simulink model "simscape_automatic_R2024a"  (R2024a)
settings: Solver=ode15s  StartTime=0.0  StopTime=inf  FixedStep=timestep
values from neighbouring files (symbols this model uses):
  timestep = 0.5    [design_details.m]
undefined symbols (not defined in the file or in its folder): CONNECTED, DEFUEL_MODE, DISCONNECT, DISCONNECTED, REFUEL_MODE
settings Model: PacingRate=0.100000  TunableVars=AC_mode_data,AC_tank_cross_sectional_area,AC_tank_radius,AC_tank_surface_area,AC_tank_vol_limit,AC_tank_volume,AC_tank_weight,AC_wall_thickness,Ambient_temp,Equivalent_battery_mass,GH2_conductivity,Generator_efficiency,H2Tables,H2_energy_density,Initial_AC_LH2_frac,Initial_AC_Tank_Gas_Temp,Initial_AC_Tank_Liquid_Temp,Initial_AC_tank_pressure,Initial_temp,LH2_conductivity,LH2_density,LH2_density_table,Required_energy,Temp_vector,engine_feed_pipe_inner_area,engine_feed_pipe_inner_diameter,engine_feed_pipe_outer_area,engine_feed_pipe_outer_diameter,engine_feed_valve_discharge_ratio,engine_feed_valve_orifice_area,engine_feed_valve_orifice_radius,hose_length,hose_thermal_conductivity,initial_hose_p,liquid_supply_SOV_leak_frac,m_LH2,mass_flow_rate,mass_per_length_engine_feed,mass_per_length_return,mass_per_length_supply,max_pressure,max_stress,phase,pipe_thermal_conductivity,pressure_vector,radiation_constant,refuel_time,return_pipe_inner_area,return_pipe_inner_diameter,return_pipe_outer_area,return_pipe_outer_diameter,return_valve_discharge_ratio,return_valve_orifice_area,return_valve_orifice_radius,short_pressure_vector,short_temp_vector,steel_conductivity,steel_density,steel_emmissitivity,steel_heat_capacity,stopTime,supply_pipe_inner_area,supply_pipe_inner_diameter,supply_pipe_outer_area,supply_pipe_outer_diameter,supply_valve_discharge_ratio,supply_valve_orifice_area,supply_valve_orifice_radius,time_array,timestep,u_max_gas,u_min_liquid,valve_diameter_vector,valve_laminar_p_ratio,wall_thickness,AC_return_valve_discharge_coeff,AC_return_valve_inner_diameter,AC_return_valve_laminar_p_ratio,AC_return_valve_leakage,AC_return_valve_orifice_area,AC_return_valve_port_inner_area,AC_return_valve_port_inner_diameter,AC_supply_valve_discharge_coeff,AC_supply_valve_inner_diameter,AC_supply_valve_laminar_p_ratio,AC_supply_valve_leakage,AC_supply_valve_orifice_area,AC_supply_valve_port_inner_area,AC_supply_valve_port_inner_diameter,GS_return_valve_discharge_coeff,GS_return_valve_inner_diameter,GS_return_valve_laminar_p_ratio,GS_return_valve_leakage,GS_return_valve_orifice_area,GS_return_valve_port_inner_area,GS_return_valve_port_inner_diameter,GS_supply_valve_discharge_coeff,GS_supply_valve_inner_diameter,GS_supply_valve_laminar_p_ratio,GS_supply_valve_leakage,GS_supply_valve_orifice_area,GS_supply_valve_port_inner_area,GS_supply_valve_port_inner_diameter,LH2_prop_valve_discharge_coeff,LH2_prop_valve_inner_diameter,LH2_prop_valve_laminar_p_ratio,LH2_prop_valve_leakage,LH2_prop_valve_orifice_area,LH2_prop_valve_port_inner_area,LH2_prop_valve_port_inner_diameter,Return_gas_prop_valve_discharge_coeff,Return_gas_prop_valve_inner_diameter,Return_gas_prop_valve_laminar_p_ratio,Return_gas_prop_valve_leakage,Return_gas_prop_valve_orifice_area,Return_gas_prop_valve_port_inner_area,Return_gas_prop_valve_port_inner_diameter,return_coupling_discharge_coeff,return_coupling_port_inner_area,return_coupling_port_inner_diameter,return_coupling_valve_inner_diameter,return_coupling_valve_laminar_p_ratio,return_coupling_valve_leakage,return_coupling_valve_orifice_area,supply_coupling_discharge_coeff,supply_coupling_port_inner_area,supply_coupling_port_inner_diameter,supply_coupling_valve_inner_diameter,supply_coupling_valve_laminar_p_ratio,supply_coupling_valve_leakage,supply_coupling_valve_orifice_area,AC_bypass_line_port_inner_area,AC_bypass_line_port_inner_diameter,AC_bypass_line_port_outer_diameter,AC_bypass_pipe_length,AC_engine_feed_pipe_length,AC_engine_feed_port_inner_area,AC_engine_feed_port_inner_diameter,AC_engine_feed_port_outer_diameter,AC_engine_valve_discharge_coeff,AC_engine_valve_inner_diameter,AC_engine_valve_laminar_p_ratio,AC_engine_valve_leakage,AC_engine_valve_orifice_area,AC_return_line_port_inner_area,AC_return_line_port_inner_diameter,AC_return_line_port_outer_diameter,AC_return_pipe_length,AC_supply_line_port_inner_area,AC_supply_line_port_inner_diameter,AC_supply_line_port_outer_diameter,AC_supply_pipe_length,AC_vent_line_port_inner_area,AC_vent_line_port_inner_diameter,AC_vent_valve_discharge_coeff,AC_vent_valve_orifice_area,AC_vent_valve_orifice_inner_diameter,Gas_prop_valve_discharge_coeff,Gas_prop_valve_inner_diameter,Gas_prop_valve_laminar_p_ratio,Gas_prop_valve_leakage,Gas_prop_valve_orifice_area,mass_per_length_bypass,return_valve_orifice_diameter,supply_valve_orifice_diameter,thermal_mass_per_length_bypass,thermal_mass_per_length_engine_feed,thermal_mass_per_length_return,thermal_mass_per_length_supply,ABORT_MODE,AC_tank_liquid_heat_transfer_coeff,AC_tank_vapour_heat_transfer_coeff,CHILLDOWN,CLOSE,CONNECTED,DEFUEL,DEFUEL_MODE,DISCONNECT,DISCONNECTED,FEED,GS_vent_cracking_delta_P,GS_vent_discharge_coeff,GS_vent_open_delta_P,Gas_prop_valve_gain,Gas_prop_valve_stroke,IDLE,LH2_prop_valve_gain,LH2_prop_valve_stroke,OPEN,OVEREFILL,PID_timestep,REFUEL,REFUEL_MODE,Return_gas_prop_valve_gain,Return_gas_prop_valve_min_open,Return_gas_prop_valve_stroke,WARMUP,i,tf_delay,vent_tf_delay  TunableVarsStorageClass=Auto,Auto,Auto,Auto,Auto,Auto,Auto,Auto,Auto,Auto,Auto,Auto,Auto,Auto,Auto,Auto,Auto,Auto,Auto,Auto,Auto,Auto,Auto,Auto,Auto,Auto,Auto,Auto,Auto,Auto,Auto,Auto,Auto,Auto,Auto,Auto,Auto,Auto,Auto,Auto,Auto,Auto,Auto,Auto,Auto,Auto,Auto,Auto,Auto,Auto,Auto,Auto,Auto,Auto,Auto,Auto,Auto,Auto,Auto,Auto,Auto,Auto,Auto,Auto,Auto,Auto,Auto,Auto,Auto,Auto,Auto,Auto,Auto,Auto,Auto,Auto,Auto,Auto,Auto,Auto,Auto,Auto,Auto,Auto,Auto,Auto,Auto,Auto,Auto,Auto,Auto,Auto,Auto,Auto,Auto,Auto,Auto,Auto,Auto,Auto,Auto,Auto,Auto,Auto,Auto,Auto,Auto,Auto,Auto,Auto,Auto,Auto,Auto,Auto,Auto,Auto,Auto,Auto,Auto,Auto,Auto,Auto,Auto,Auto,Auto,Auto,Auto,Auto,Auto,Auto,Auto,Auto,Auto,Auto,Auto,Auto,Auto,Auto,Auto,Auto,Auto,Auto,Auto,Auto,Auto,Auto,Auto,Auto,Auto,Auto,Auto,Auto,Auto,Auto,Auto,Auto,Auto,Auto,Auto,Auto,Auto,Auto,Auto,Auto,Auto,Auto,Auto,Auto,Auto,Auto,Auto,Auto,Auto,Auto,Auto,Auto,Auto,Auto,Auto,Auto,Auto,Auto,Auto,Auto,Auto,Auto,Auto,Auto,Auto,Auto,Auto,Auto,Auto,Auto,Auto,Auto,Auto,Auto,Auto,Auto  TunableVarsTypeQualifier=,,,,,,,,,,,,,,,,,,,,,,,,,,,,,,,,,,,,,,,,,,,,,,,,,,,,,,,,,,,,,,,,,,,,,,,,,,,,,,,,,,,,,,,,,,,,,,,,,,,,,,,,,,,,,,,,,,,,,,,,,,,,,,,,,,,,,,,,,,,,,,,,,,,,,,,,,,,,,,,,,,,,,,,,,,,,,,,,,,,,,,,,,,,,,,,,,,,,,,,  Creator=MW  LastModifiedBy=MW
settings SolverCC: MaxConsecutiveMinStep=3  DaesscMode=Robust  SolverResetMethod=Robust
settings DataIOCC: ReturnWorkspaceOutputsName=tpe7319d77_74b4_4e39_b21d_406e30cb87cb
settings ModelReferenceCC: UpdateModelReferenceTargets=IfOutOfDate
settings SFSimCC: SFSimEcho=off  SimTargetLang=C++  GPUAcceleration=on  SimDLTargetLibrary=cudnn
settings SimscapeCC: SimscapeNominalValues="[{\"value\":\"1\",\"unit\":\"A\"},{\"value\":\"0.3\",\"unit\":\"bar\"},{\"value\":\"1\",\"unit\":\"cm^2\"},{\"value\":\"1\",\"unit\":\"cm^3/s\"},{\"value\":\"1\",\"unit\":\"kJ/kg\"},{\"value\":\"1\",\"unit\":\"kW\"},{\"value\":\"1\",\"unit\":\"l\"},{\"value\":\"1\",\"unit\":\"N\"},{\"value\":\"1\",\"unit\":\"N*m\"},{\"value\":\"1\",\"unit\":\"V\"}]"  SimscapeLogType=all  SimscapeLogSimulationStatistics=on  SimscapeLogLimitData=off

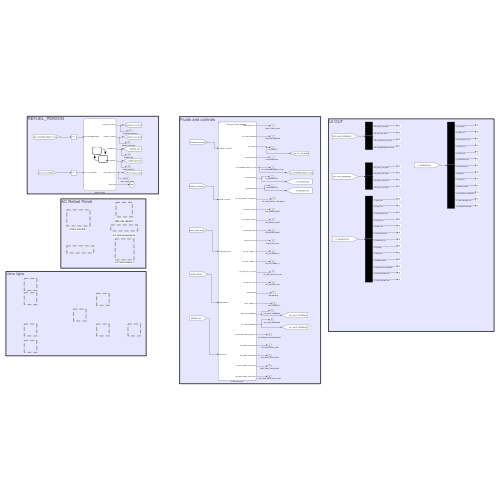
[thumbnail: Simulink's stored preview of the top-level diagram]
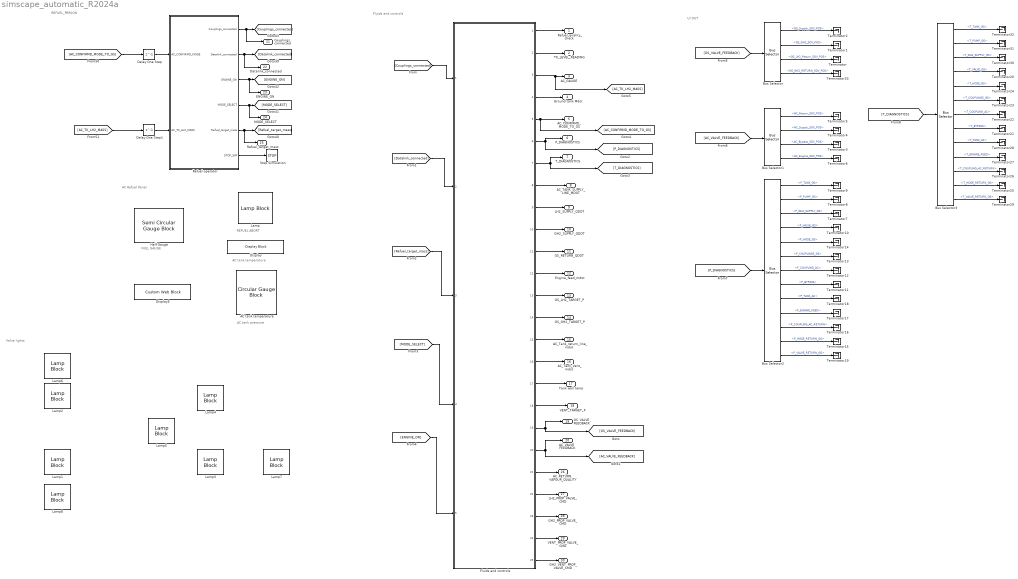
== system simscape_automatic_R2024a ==
  note: REFUEL ABORT
  note: AC tank pressure
  note: AC Refuel Panel
  note: AC tank temperature
  note: REFUEL_PERSON
  note: FUEL GAUGE
  note: UI OUT
  note: Valve lights
  note: Fluids and controls
  AC tank temperature : CircularGaugeBlock  LabelPosition=Hide  ScaleMax=0.7
  Bus Selector : BusSelector  OutputSignals=GS_Supply_SOV_POS,GS_GH2_SOV_POS,GS_LH2_Return_SOV_POS,GS_GH2_RETURN_SOV_POS
  Bus Selector1 : BusSelector  OutputSignals=AC_Return_SOV_POS,AC_Supply_SOV_POS,AC_Bypass_SOV_POS,AC_Engine_SOV_POS
  Bus Selector2 : BusSelector  OutputSignals=P_TANK_GS,P_PUMP_GS,P_GH2_SUPPLY_GS,P_VALVE_GS,P_HOSE_GS,P_COUPLINGS_GS,P_COUPLING_AC,P_BYPASS,P_TANK_AC,P_ENGINE_FEED,P_COUPLING_AC_RETURN,P_HOSE_RETURN_GS,P_VALVE_RETURN_GS
  Bus Selector3 : BusSelector  OutputSignals=T_TANK_GS,T_PUMP_GS,T_GH2_SUPPLY_GS,T_VALVE_GS,T_HOSE_GS,T_COUPLINGS_GS,T_COUPLING_AC,T_BYPASS,T_TANK_AC,T_ENGINE_FEED,T_COUPLING_AC_RETURN,T_HOSE_RETURN_GS,T_VALVE_RETURN_GS
  Delay One Step : Delay  DelayLength=1
  Delay One Step1 : Delay  DelayLength=1
  Display : DisplayBlock  LabelPosition=Hide  Transparency=1
  Display5 : CustomWebBlock  LabelPosition=Hide  ShowInitialText=on  Configuration="{\"components\":[{\"name\":\"DisplayComponent\",\"settings\":{\"bold\":false,\"font\":\"DSEG7 Classic\",\"fontColor\":[255,255,200],\"fontSize\":\"14\",\"format\":\"short\",\"formatString\":\"%d\",\"italic\":false,\"position\":[0,0,1,1],\"underline\":false}},{\"name\":\"BackgroundImageComponent\",\"settings\":{\"image\":{\"size\":[300,80],\"src\":\"data:image\\/svg+xml;base64,PHN2ZyBpZD0iZnJhbWUiIHhtbG5zPSJodHRwOi8vd3d3LnczLm9yZy8yMDAwL3N2ZyIgeG1sbnM6eGxpbms9Imh0dHA6Ly93d3cudzMub3JnLzE5OTkveGxpbmsiIHZpZXdCb3g9IjAgMCAzODAgMTAxIj48ZGVmcz48c3R5bGU+LmNscy0xe2ZpbGw6IzAwMmI0Mjt9LmNscy0ye2ZpbGw6IzQyNzA4Mjt9LmNscy0ze2ZpbGw6dXJsKCNyYWRpYWwtZ3JhZGllbnQpO308L3N0eWxlPjxyYWRpYWxHcmFkaWVudCBpZD0icmFkaWFsLWdyYWRpZW50IiBjeD0iMTkwIiBjeT0iNTAuNSIgcj0iMjY5LjIxIiBncmFkaWVudFVuaXRzPSJ1c2VyU3BhY2VPblVzZSI+PHN0b3Agb2Zmc2V0PSIwLjAxIiBzdG9wLWNvbG9yPSIjM2U0ZjU4Ii8+PHN0b3Agb2Zmc2V0PSIwLjA2IiBzdG9wLWNvbG9yPSIjNDQ1NzYxIi8+PHN0b3Agb2Zmc2V0PSIwLjE1IiBzdG9wLWNvbG9yPSIjNTU2YTc2Ii8+PHN0b3Agb2Zmc2V0PSIwLjI1IiBzdG9wLWNvbG9yPSIjNmQ4ODk1Ii8+PHN0b3Agb2Zmc2V0PSIwLjM4IiBzdG9wLWNvbG9yPSIjOGZiMmMzIi8+PHN0b3Agb2Zmc2V0PSIwLjUyIiBzdG9wLWNvbG9yPSIjYjZlNGZhIi8+PHN0b3Agb2Zmc2V0PSIxIiBzdG9wLWNvbG9yPSIjMTU0NjU3Ii8+PC9yYWRpYWxHcmFkaWVudD48L2RlZnM+PGcgaWQ9IkxheWVyXzIiIGRhdGEtbmFtZT0iTGF5ZXIgMiI+PGcgaWQ9IkxheWVyXzEtMiIgZGF0YS1uYW1lPSJMYXllciAxLTIiPjxyZWN0IGlkPSJyZWN0MTAzNiIgY2xhc3M9ImNscy0xIiB4PSIxMSIgeT0iMTEiIHdpZHRoPSIzNTgiIGhlaWdodD0iNzkiLz48cGF0aCBpZD0icGF0aDEwMzgiIGNsYXNzPSJjbHMtMiIgZD0iTTgsOFY5M0gzNzJWOFpNMzY5LDkwSDExVjExSDM2OVoiLz48cGF0aCBpZD0icGF0aDEwNDAiIGNsYXNzPSJjbHMtMyIgZD0iTTAsMFYxMDFIMzgwVjBaTTM3Miw5M0g4VjhIMzcyWiIvPjwvZz48L2c+PC9zdmc+\",\"srcOrientation\":\"Right\"},\"position\":[0,0,1,1],\"scaleMode\":\"0\"}},{\"name\":\"ForegroundImageComponent\",\"settings\":{\"angle\":0,\"image\":{\"size\":[0,0],\"src\":\"default\"},\"isForeground\":1,\"position\":[0,0,1,1],\"scaleMode\":\"0\"}}],\"settings\":{\"BindingType\":\"signal\",\"aspectRatio\":1.032258064516129,\"backgroundColor\":[0,0,0,\"1\"],\"backgroundOffset\":0.14,\"backgroundOpacity\":1,\"fixedAspectRatio\":\"on\",\"showBackgroundColor\":false,\"value\":0,\"version\":\"R2023b\"},\"type\":\"Display\"}"
  Fluids and controls : Subsystem  ReferencedSubsystem=fluids_and_control_subsystem
  Half Gauge : SemiCircularGaugeBlock  ScaleMax=35
  Lamp{,1..8} (9 alike) : LampBlock  LabelPosition=Hide
  Refuel operator : Stateflow chart  TreatAsAtomicUnit=on  SystemSampleTime=timestep
  Stop Simulation : Stop
  Terminator{,1..33} (34 alike) : Terminator
  Refuel_quality_check : Outport
  TK_LEVEL_READING : Outport  Port=2
  AC_GAUGE : Outport  Port=3
  Ground tank Mdot : Outport  Port=4
  AC_CONFIRMD_MODE_TO_GS : Outport  Port=5
  P_DIAGNOSTICS : Outport  Port=6
  T_DIAGNOSTICS : Outport  Port=7
  AC_TANK_SUPPLY_LINE_MDOT : Outport  Port=8
  LH2_SUPPLY_QDOT : Outport  Port=9
  GH2_SUPPLY_QDOT : Outport  Port=10
  GS_RETURN_QDOT : Outport  Port=11
  Engine_feed_mdot : Outport  Port=12
  GS_LH2_TARGET_P : Outport  Port=13
  GS_GH2_TARGET_P : Outport  Port=14
  AC_Tank_return_line_mdot : Outport  Port=15
  AC_Tank_Vent_mdot : Outport  Port=16
  Tank wall temp : Outport  Port=17
  VENT_TARGET_P : Outport  Port=18
  GS_VALVE_FEEDBACK : Outport  Port=19
  AC_VALVE_FEEDBACK : Outport  Port=20
  Couplings_connected : Outport  Port=21
  Datalink_connected : Outport  Port=22
  ENGINE_ON : Outport  Port=23
  MODE_SELECT : Outport  Port=24
  Refuel_target_mass : Outport  Port=25
  AC_RETURN_VAPOUR_QUALITY : Outport  Port=26
  LH2_PROP_VALVE_CMD : Outport  Port=27
  GH2_PROP_VALVE_CMD : Outport  Port=28
  VENT_PROP_VALVE_CMD : Outport  Port=29
  GH2_VENT_PROP_VALVE_CMD : Outport  Port=30
  wires:
  Refuel operator/1(Couplings_connected) -> Couplings_connected/1, [Couplings_connected]
  Refuel operator/2(Datalink_connected) -> Datalink_connected/1, [Datalink_connected]
  Refuel operator/4(MODE_SELECT) -> MODE_SELECT/1, [MODE_SELECT]
  Refuel operator/3(ENGINE_ON) -> ENGINE_ON/1, [ENGINE_ON]
  Refuel operator/5(Refuel_target_mass) -> Refuel_target_mass/1, [Refuel_target_mass]
  [AC_CONFIRMD_MODE_TO_GS] -> Delay One Step/1
  Delay One Step/1 -> Refuel operator/1(AC_CONFIRMD_MODE)
  [AC_TK_LH2_MASS] -> Delay One Step1/1
  Delay One Step1/1 -> Refuel operator/2(AC_TK_LH2_MASS)
  Refuel operator/6(STOP_SIM) -> Stop Simulation/1
  [T_DIAGNOSTICS] -> Bus Selector3/1
  Bus Selector3/3 -> Terminator30/1  "<T_GH2_SUPPLY_GS>"
  Bus Selector/1 -> Terminator2/1  "<GS_Supply_SOV_POS>"
  Bus Selector3/2 -> Terminator31/1  "<T_PUMP_GS>"
  Bus Selector3/12 -> Terminator25/1  "<T_HOSE_RETURN_GS>"
  Bus Selector2/9 -> Terminator18/1  "<P_TANK_AC>"
  Bus Selector3/11 -> Terminator26/1  "<T_COUPLING_AC_RETURN>"
  Bus Selector3/4 -> Terminator20/1  "<T_VALVE_GS>"
  Bus Selector/3 -> Terminator/1  "<GS_LH2_Return_SOV_POS>"
  Bus Selector3/5 -> Terminator24/1  "<T_HOSE_GS>"
  Bus Selector3/6 -> Terminator23/1  "<T_COUPLINGS_GS>"
  [GS_VALVE_FEEDBACK] -> Bus Selector/1
  Bus Selector2/5 -> Terminator14/1  "<P_HOSE_GS>"
  Bus Selector2/3 -> Terminator7/1  "<P_GH2_SUPPLY_GS>"
  Bus Selector1/1 -> Terminator5/1  "<AC_Return_SOV_POS>"
  Bus Selector2/7 -> Terminator12/1  "<P_COUPLING_AC>"
  Bus Selector3/9 -> Terminator28/1  "<T_TANK_AC>"
  Bus Selector3/1 -> Terminator32/1  "<T_TANK_GS>"
  Bus Selector2/13 -> Terminator19/1  "<P_VALVE_RETURN_GS>"
  Bus Selector3/10 -> Terminator27/1  "<T_ENGINE_FEED>"
  Bus Selector2/12 -> Terminator15/1  "<P_HOSE_RETURN_GS>"
  Bus Selector1/4 -> Terminator6/1  "<AC_Engine_SOV_POS>"
  Bus Selector2/6 -> Terminator13/1  "<P_COUPLINGS_GS>"
  [P_DIAGNOSTICS] -> Bus Selector2/1
  Bus Selector2/4 -> Terminator10/1  "<P_VALVE_GS>"
  Bus Selector2/11 -> Terminator16/1  "<P_COUPLING_AC_RETURN>"
  Bus Selector3/13 -> Terminator29/1  "<T_VALVE_RETURN_GS>"
  Bus Selector2/2 -> Terminator8/1  "<P_PUMP_GS>"
  [AC_VALVE_FEEDBACK] -> Bus Selector1/1
  Bus Selector1/2 -> Terminator4/1  "<AC_Supply_SOV_POS>"
  Bus Selector/2 -> Terminator1/1  "<GS_GH2_SOV_POS>"
  Bus Selector1/3 -> Terminator3/1  "<AC_Bypass_SOV_POS>"
  Bus Selector2/8 -> Terminator11/1  "<P_BYPASS>"
  Bus Selector3/7 -> Terminator22/1  "<T_COUPLING_AC>"
  Bus Selector2/10 -> Terminator17/1  "<P_ENGINE_FEED>"
  Bus Selector2/1 -> Terminator9/1  "<P_TANK_GS>"
  Bus Selector3/8 -> Terminator21/1  "<T_BYPASS>"
  Fluids and controls/6 -> P_DIAGNOSTICS/1, [P_DIAGNOSTICS]
  Fluids and controls/16 -> AC_Tank_Vent_mdot/1
  Fluids and controls/3 -> [AC_TK_LH2_MASS], AC_GAUGE/1
  [Datalink_connected] -> Fluids and controls/2
  Fluids and controls/9 -> LH2_SUPPLY_QDOT/1
  Fluids and controls/11 -> GS_RETURN_QDOT/1
  Fluids and controls/2 -> TK_LEVEL_READING/1
  Fluids and controls/5 -> [AC_CONFIRMD_MODE_TO_GS], AC_CONFIRMD_MODE_TO_GS/1
  Fluids and controls/18 -> VENT_TARGET_P/1
  Fluids and controls/1 -> Refuel_quality_check/1
  Fluids and controls/14 -> GS_GH2_TARGET_P/1
  Fluids and controls/17 -> Tank wall temp/1
  [Refuel_target_mass] -> Fluids and controls/3
  Fluids and controls/13 -> GS_LH2_TARGET_P/1
  [Couplings_connected] -> Fluids and controls/1
  [ENGINE_ON] -> Fluids and controls/5
  Fluids and controls/19 -> GS_VALVE_FEEDBACK/1, [GS_VALVE_FEEDBACK]
  Fluids and controls/10 -> GH2_SUPPLY_QDOT/1
  Fluids and controls/20 -> AC_VALVE_FEEDBACK/1, [AC_VALVE_FEEDBACK]
  Fluids and controls/8 -> AC_TANK_SUPPLY_LINE_MDOT/1
  Fluids and controls/7 -> T_DIAGNOSTICS/1, [T_DIAGNOSTICS]
  Fluids and controls/12 -> Engine_feed_mdot/1
  [MODE_SELECT] -> Fluids and controls/4
  Fluids and controls/15 -> AC_Tank_return_line_mdot/1
  Fluids and controls/4 -> Ground tank Mdot/1
  Fluids and controls/21 -> AC_RETURN_VAPOUR_QUALITY/1
  Fluids and controls/22 -> LH2_PROP_VALVE_CMD/1
  Fluids and controls/23 -> GH2_PROP_VALVE_CMD/1
  Fluids and controls/24 -> VENT_PROP_VALVE_CMD/1
  Bus Selector/4 -> Terminator33/1  "<GS_GH2_RETURN_SOV_POS>"
  Fluids and controls/25 -> GH2_VENT_PROP_VALVE_CMD/1

== stateflow chart simscape_automatic_R2024a/Refuel operator ==
  state STANDBY
    en:
    STOP_SIM = false;
  state START_WARM_TANK_REFUEL
    en:
    Couplings_connected = CONNECTED;
    Datalink_connected = CONNECTED;
    Refuel_target_mass = 28.2;
    MODE_SELECT = REFUEL_MODE;
    ENGINE_ON = false;
  state WAIT_WARMUP
  state FLIGHT
    en:
    Couplings_connected = DISCONNECTED;
    Datalink_connected = DISCONNECTED;
    ENGINE_ON = true;
  state START_COLD_TANK_REFUEL1
    en:
    Couplings_connected = CONNECTED;
    Datalink_connected = CONNECTED;
    Refuel_target_mass = 28.2;
    MODE_SELECT = REFUEL_MODE;
    ENGINE_ON = false;
  state WAIT_WARMUP1
  state READY_DEFUEL
    en:
    Couplings_connected = DISCONNECTED;
    Datalink_connected = DISCONNECTED;
    ENGINE_ON = false;
  state START_COLD_TANK_DEFUEL
    en:
    Couplings_connected = CONNECTED;
    Datalink_connected = CONNECTED;
    Refuel_target_mass = 0;
    MODE_SELECT = DEFUEL_MODE;
    ENGINE_ON = false;
  state WAIT_WARMUP2
  state SET_COMPLETE
    en:
    STOP_SIM = true;
  (default) -> STANDBY
  STANDBY -> START_WARM_TANK_REFUEL : after(10, sec)
  START_WARM_TANK_REFUEL -> WAIT_WARMUP : [AC_TK_LH2_MASS >= Refuel_target_mass]
  WAIT_WARMUP -> FLIGHT : [AC_CONFIRMD_MODE == DISCONNECT]
  FLIGHT -> START_COLD_TANK_REFUEL1 : [AC_TK_LH2_MASS  < 1]
  START_COLD_TANK_REFUEL1 -> WAIT_WARMUP1 : [AC_TK_LH2_MASS >= Refuel_target_mass]
  WAIT_WARMUP1 -> READY_DEFUEL : [AC_CONFIRMD_MODE == DISCONNECT]
  READY_DEFUEL -> START_COLD_TANK_DEFUEL : after(10, sec)
  START_COLD_TANK_DEFUEL -> WAIT_WARMUP2
  WAIT_WARMUP2 -> SET_COMPLETE : [AC_CONFIRMD_MODE == DISCONNECT]
  data: Couplings_connected output boolean; Datalink_connected output boolean; ENGINE_ON output boolean; MODE_SELECT output boolean; Refuel_target_mass output double; CONNECTED parameter; REFUEL_MODE parameter; AC_CONFIRMD_MODE input; DISCONNECTED parameter; AC_TK_LH2_MASS input; DISCONNECT parameter; STOP_SIM output; DEFUEL_MODE parameter
